simulink model "modelo_resorte"  (R2022b)
settings: Solver=VariableStepAuto  StartTime=0.0  StopTime=200  RelTol=1e-3
values from neighbouring files (symbols this model uses):
  m1 = 1    [din.mat]    (also in matlab.mat = 1.58160160615)
  m2 = 1    [din.mat]    (also in matlab.mat = 1.16504377885)
settings Model: Creator=adanaviles  LastModifiedBy=adanaviles

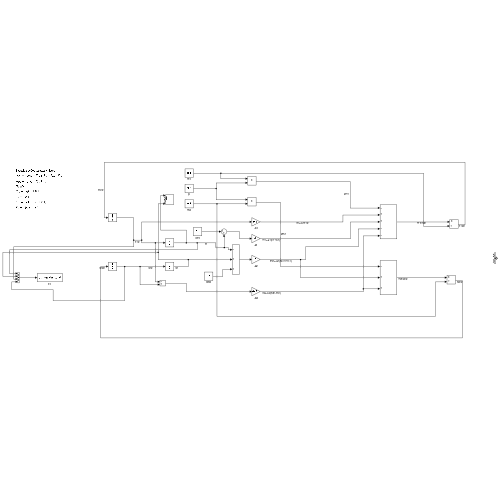
[thumbnail: Simulink's stored preview of the top-level diagram]
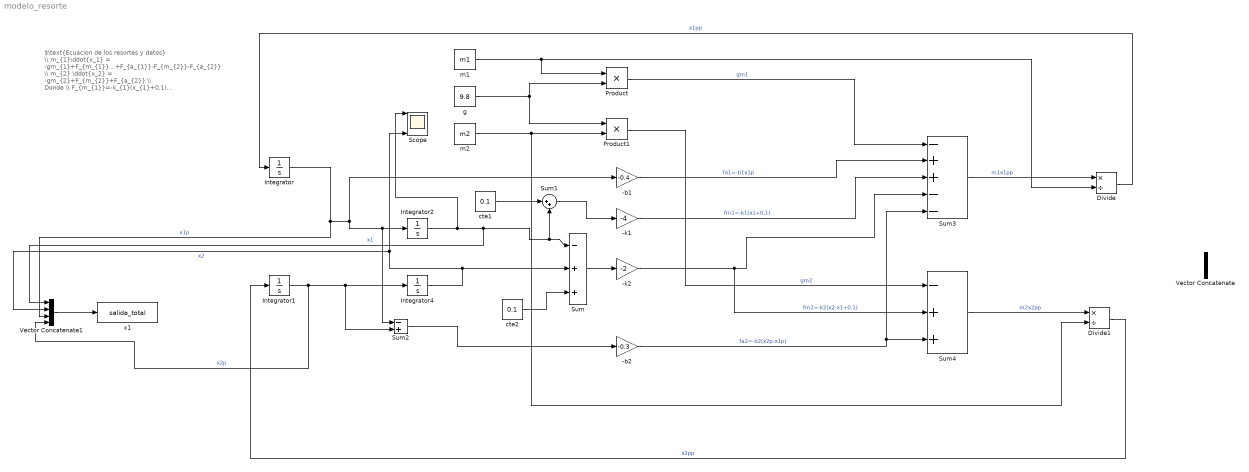
== system modelo_resorte ==
  note: $\text{Ecuacion de los resortes y datos} \\ m_{1}\ddot{x_1} = -gm_{1}+F_{m_{1}}+F_{a_{1}}-F_{m_{2}}-F_{a_{2}} \\ m_{2} \ddot{x_2} = -gm_{2}+F_{m_{2}}+F_{a_{2}} \\ Donde \\ F_{m_{1}}=-k_{1}(x_{1}+0,1) \\ F_{a_{1}}=-b_{1}\dot{x_{1}} \\ F_{m_{2}}=-k_{2}(x_{2}-x_{1}+0,1) \\ F_{a_{2}}=-b_{2}(\dot{x_{2}} -\dot{x_{1}})$
  -b1 : Gain  Gain=-0.4
  -b2 : Gain  Gain=-0.3
  -k1 : Gain  Gain=-4
  -k2 : Gain  Gain=-2
  Divide : Product  Inputs=*/
  Divide1 : Product  Inputs=*/
  Integrator : Integrator
  Integrator1 : Integrator
  Integrator2 : Integrator  InitialCondition=-0.1
  Integrator4 : Integrator  InitialCondition=-0.23
  Product : Product
  Product1 : Product
  Scope : Scope  NumInputPorts=4
  Sum : Sum  Inputs=-++
  Sum1 : Sum  Inputs=|++
  Sum2 : Sum  Inputs=-+
  Sum3 : Sum  Inputs=-++--
  Sum4 : Sum  Inputs=-++
  Vector Concatenate : Concatenate
  Vector Concatenate1 : Concatenate  NumInputs=4  ConcatenateDimension=4
  cte1 : Constant  Value=0.1
  cte2 : Constant  Value=0.1
  g : Constant  Value=9.8
  m1 : Constant  Value=m1
  m2 : Constant  Value=m2
  x1 : ToWorkspace  VariableName=salida_total  SampleTime=-1
  wires:
  Integrator/1 -> Vector Concatenate1/3, Sum2/1, Integrator2/1, -b1/1  "x1p"
  Integrator1/1 -> Integrator4/1, Sum2/2, Vector Concatenate1/4  "x2p"
  Divide/1 -> Integrator/1  "x1pp"
  Integrator2/1 -> Scope/1, Vector Concatenate1/1, Sum1/2, Sum/1  "x1"
  Integrator4/1 -> Vector Concatenate1/2, Scope/4, Sum/2  "x2"
  g/1 -> Product1/1, Product/2
  Product/1 -> Sum3/1  "gm1"
  Product1/1 -> Sum4/1  "gm2"
  -b1/1 -> Sum3/2  "fa1=-b1x1p"
  cte2/1 -> Sum/3
  Sum/1 -> -k2/1
  -k2/1 -> Sum4/2, Sum3/4  "fm2=-k2(x2-x1+0.1)"
  cte1/1 -> Sum1/1
  Sum1/1 -> -k1/1
  -k1/1 -> Sum3/3  "fm1=-k1(x1+0,1)"
  Sum2/1 -> -b2/1
  -b2/1 -> Sum4/3, Sum3/5  "fa2=-b2(x2p-x1p)"
  Sum3/1 -> Divide/1  "m1x1pp"
  m1/1 -> Divide/2, Product/1
  m2/1 -> Divide1/2, Product1/2
  Sum4/1 -> Divide1/1  "m2x2pp"
  Divide1/1 -> Integrator1/1  "x2pp"
  Vector Concatenate1/1 -> x1/1
